simulink model "laneChange3"  (R2017a)
settings: Solver=VariableStepAuto  StartTime=0  StopTime=10  MaxStep=0.05  RelTol=1e-3
model workspace (MAT data in the model file):
  FARAWAY = Simulink.Parameter
  FARAWAY.Value = 100
  FARAWAY.DataType = 'auto'
  FARAWAY.Dimensions = [1 1]
  LANE_NUM = 2
  LANE_WIDTH = 1
  MIN_SAFE_DIST = Simulink.Parameter
  MIN_SAFE_DIST.Value = 1
  MIN_SAFE_DIST.DataType = 'auto'
  MIN_SAFE_DIST.Dimensions = [1 1]
  ROAD_WIDTH = 2
  SAFE_FACTOR = Simulink.Parameter
  SAFE_FACTOR.Value = 0.25
  SAFE_FACTOR.DataType = 'auto'
  SAFE_FACTOR.Dimensions = [1 1]
  WORLD_SIZE = 12
  dt = Simulink.Parameter
  dt.Value = 0.05
  dt.DataType = 'auto'
  dt.Dimensions = [1 1]
undefined symbols (not defined in the file or in its folder): m, n
(part 1 of 2)
settings Model: Creator=larry  LastModifiedBy=larry

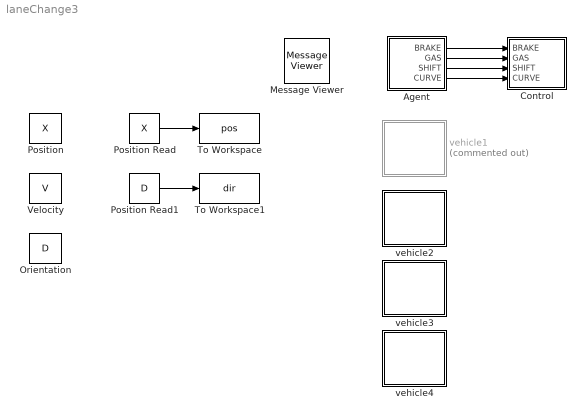
== system laneChange3 ==
  Agent : Stateflow chart  TreatAsAtomicUnit=on
  Control : Stateflow chart  TreatAsAtomicUnit=on
  Message Viewer : MessageViewer
  Orientation : DataStoreMemory  DataStoreName=D  WriteAfterReadMsg=warning  InitialValue=[1 1 1 1;0 0 0 0]  ShowAdditionalParam=off  OutDataTypeStr=double
  Position : DataStoreMemory  DataStoreName=X  InitialValue=[-11 -11 -9 11;-0.5 0.5 0.5 0.5]  ShowAdditionalParam=off  OutDataTypeStr=double
  Position Read : DataStoreRead  DataStoreName=X
  Position Read1 : DataStoreRead  DataStoreName=D
  To Workspace : ToWorkspace  VariableName=pos  SampleTime=-1
  To Workspace1 : ToWorkspace  VariableName=dir  SampleTime=-1
  Velocity : DataStoreMemory  DataStoreName=V  InitialValue=[0 0 0 0;0 0 0 0]  ShowAdditionalParam=off  OutDataTypeStr=double
  vehicle1 : Stateflow chart  Commented=on  TreatAsAtomicUnit=on
  vehicle2 : Stateflow chart  TreatAsAtomicUnit=on
  vehicle3 : Stateflow chart  TreatAsAtomicUnit=on
  vehicle4 : Stateflow chart  TreatAsAtomicUnit=on
  wires:
  Position Read/1 -> To Workspace/1
  Agent/2(GAS) -> Control/2(GAS)
  Agent/1(BRAKE) -> Control/1(BRAKE)
  Agent/3(SHIFT) -> Control/3(SHIFT)
  Agent/4(CURVE) -> Control/4(CURVE)
  Position Read1/1 -> To Workspace1/1

== stateflow chart laneChange3/vehicle2 ==
  state Straight
    en:
    safeDist = max(norm(V(:,this))*SAFE_FACTOR,MIN_SAFE_DIST);
    du:
    safeDist = max(norm(V(:,this))*SAFE_FACTOR,MIN_SAFE_DIST);
    state Follow
      en:
      [dxfr, dvfr] = frontCarInfo();
      du:
      [dxfr, dvfr] = frontCarInfo();
      state Safe
        du:
        if dvfr < 0
        accelerateDrive();
        else
        slowDownDrive();
        end
      state Dangerous
        du:
        slowDownDrive();
      Safe -> Dangerous : [dxfr < 1*safeDist]
      Dangerous -> Safe : [dxfr > 1.5*safeDist]
      (default) -> Dangerous [order 2]
      (default) -> Safe [order 1] : [dxfr > 1.5*safeDist]
    state FreeDriving
      state Accelerate
        du:
        accelerateDrive();
      state FixRate
        en:
        setRateTo(V_MAX);
        du:
        fixedRateDrive();
      (default) -> Accelerate [order 2]
      Accelerate -> FixRate : [reach(V_MAX)]
      (default) -> FixRate [order 1] : [reach(V_MAX)]
    (default) -> Follow [order 1] : [hasFrontCar()]
    (default) -> FreeDriving [order 2]
    FreeDriving -> Follow : [hasFrontCar()]
    Follow -> FreeDriving : [frontCarHasLeft()]
  data: res function_output; res function_output; res function_output; target function_input; target function_input; dx function_output; dv function_output; idx function_output; X data_store_memory; this local uint8 size=1 =uint8(2); A_MAX constant double =2.5; D data_store_memory; V_MAX constant double =1.5; V data_store_memory; MIN_SAFE_DIST parameter; WORLD_SIZE parameter; dt parameter; dxfr local; dvfr local; safeDist local; FARAWAY parameter; SAFE_FACTOR parameter
  function slowDownDrive:
    | function slowDownDrive
    |  
    | x = X(:,this);
    | v = V(:,this);
    | a = D(:,this) * (-A_MAX);
    | 
    | if isequal(v, [0;0])
    |     return;
    | end
    | 
    | x = x + v * dt + 0.5 * a * dt * dt;
    | if dot(v, v+a*dt) >= 0
    |     v = v + a * dt;
    | else
    |     v = 0 * v;
    | end
    | 
    | % a rounded world
    | if x(1) > WORLD_SIZE
    |     x(1) = -WORLD_SIZE;
    | elseif x(1) < -WORLD_SIZE
    |     x(1) = WORLD_SIZE;
    | elseif x(2) > WORLD_SIZE
    |     x(2) = -WORLD_SIZE;
    | elseif x(2) < -WORLD_SIZE
    |     x(2) = WORLD_SIZE;
    | end
    | 
    | X(:,this) = x;
    | V(:,this) = v;
  function res = hasFrontCar:
    | function res = hasFrontCar
    | 
    | % constants
    | THRES = 1.5 * safeDist;
    | RANGE = 2 * WORLD_SIZE;
    | 
    | res = false;
    | 
    | % row of X: coordinate, col of X: num of cars
    | num = size(X, 2);
    | if num == 1
    |     return;
    | end
    | 
    | dx = ones(num, 1)*FARAWAY;
    | x = X(:,this);
    | d = D(:,this);
    | carSize = [0.3; 0.4];
    | 
    | for k=1:length(dx)
    |     
    |     if k ~= this
    |         % compute difference
    |         xdelta = X(:,k) - x;
    |     
    |         % parallel and vertical distance
    |         delta_p = dot(xdelta, d);
    |         delta_v = norm(xdelta - (d * delta_p));
    |     
    |         % vertical distance is larger than car width
    |         if delta_v < carSize(1)
    |             dx(k) = delta_p;
    |       
    |             % a rounded world
    |             dx(k) = mod((dx(k)+RANGE), RANGE);
    |         end
    |     end
    | end
    | 
    | % set zero dX to a large enough value
    | closest = min(dx);
    | res = closest <= THRES;
  function res = frontCarHasLeft:
    | function res = frontCarHasLeft
    | 
    | % Constants 
    | THRES = 2.5 * safeDist;
    | RANGE = 2 * WORLD_SIZE;
    | 
    | % if only one car in the environment return directly
    | res = true;
    | num = size(X, 1);
    | if num == 1
    |     return;
    | end
    | 
    | % get the closet car index and its distance
    | dx = zeros(num, 1);
    | x = X(:,this);
    | d = D(:,this);
    | car_size = [0.3; 0.4];
    | 
    | for k=1:length(dx)
    |     
    |     xdelta = X(:,k) - x;
    |     xdelta_p = dot(xdelta, d);                  % parallel component
    |     xdelta_v = norm(xdelta - (d * xdelta_p));   % vertical component
    |     
    |     % when the vertical component is larger than the car width
    |     if xdelta_v < car_size(1)
    |         dx(k) = xdelta_p;
    |         % since we are in the round world, normalize the distance if the 
    |         % front car is behind us 
    |         % a rounded world
    |         dx(k) = mod((dx(k)+RANGE), RANGE);
    |     else
    |         dx(k) = FARAWAY;
    |     end
    | end
    | 
    | % set the zero dx to a large enough value for convenience
    | dx(dx == 0) = FARAWAY;
    | closest = min(dx);
    | res = closest > THRES;
  function res = reach(target):
    | function res = reach(target)
    | 
    | res = abs(target - norm(V(:,this))) < 0.125;
  function accelerateDrive:
    | function accelerateDrive
    | 
    | x = X(:,this);
    | v = V(:,this);
    | a = D(:,this) * A_MAX;
    | 
    | x = x + v * dt + 0.5 * a * dt * dt;
    | v = v + a * dt;
    | 
    | % a rounded world
    | if x(1) > WORLD_SIZE
    |     x(1) = -WORLD_SIZE;
    | elseif x(1) < -WORLD_SIZE
    |     x(1) = WORLD_SIZE;
    | elseif x(2) > WORLD_SIZE
    |     x(2) = -WORLD_SIZE;
    | elseif x(2) < -WORLD_SIZE
    |     x(2) = WORLD_SIZE;
    | end
    | 
    | X(:,this) = x;
    | V(:,this) = v;
  function fixedRateDrive:
    | function fixedRateDrive
    | 
    | x = X(:,this);
    | v = V(:,this);
    | 
    | % update new position
    | x = x + v * dt;
    | 
    | % a rounded world
    | if x(1) > WORLD_SIZE
    |     x(1) = -WORLD_SIZE;
    | elseif x(1) < -WORLD_SIZE
    |     x(1) = WORLD_SIZE;
    | elseif x(2) > WORLD_SIZE
    |     x(2) = -WORLD_SIZE;
    | elseif x(2) < -WORLD_SIZE
    |     x(2) = WORLD_SIZE;
    | end
    | 
    | X(:,this) = x;
  function setRateTo(target):
    | function setRateTo(target)
    | 
    | V(:,this) = D(:,this) * target;
  function [dx,dv] = frontCarInfo:
    | function [dx,dv] = frontCarInfo()
    | 
    | index = frontCarIndex();
    | 
    | x = X(:,this);
    | v = V(:,this);
    | d = D(:,this);
    | 
    | xfront = X(:,index);
    | vfront = V(:,index);
    | 
    | range = 2 * WORLD_SIZE;
    | 
    | dx = mod((dot(xfront - x, d)+range), range);
    | dv = dot(vfront-v, d);
    | 
    | end
  function idx = frontCarIndex:
    | function idx = frontCarIndex
    | 
    | RANGE = 2*WORLD_SIZE;
    | 
    | dx = ones(size(X, 2), 1)*FARAWAY;
    | x = X(:,this);
    | v = V(:,this);
    | d = D(:,this);
    | 
    | for k=1:length(dx)
    |     xk = X(:,k);
    |     if k ~= this && (abs(xk(2)-x(2)) < 1)
    |         dx(k) = dot(xk - x, d);
    |         dx(k) = mod((dx(k)+RANGE), RANGE);
    |     end
    | end
    | 
    | % set zero dx to a large enough value
    | [~, idx] = min(dx);
    | idx = uint8(idx);
    | 
    | end

== stateflow chart laneChange3/vehicle3 ==
  state Straight
    en:
    safeDist = max(norm(V(:,this))*SAFE_FACTOR,MIN_SAFE_DIST);
    du:
    safeDist = max(norm(V(:,this))*SAFE_FACTOR,MIN_SAFE_DIST);
    state Follow
      en:
      [dxfr, dvfr] = frontCarInfo();
      du:
      [dxfr, dvfr] = frontCarInfo();
      state Safe
        du:
        if dvfr < 0
        accelerateDrive();
        else
        slowDownDrive();
        end
      state Dangerous
        du:
        slowDownDrive();
      Safe -> Dangerous : [dxfr < 1*safeDist]
      Dangerous -> Safe : [dxfr > 1.5*safeDist]
      (default) -> Dangerous [order 2]
      (default) -> Safe [order 1] : [dxfr > 1.5*safeDist]
    state FreeDriving
      state Accelerate
        du:
        accelerateDrive();
      state FixRate
        en:
        setRateTo(V_MAX);
        du:
        fixedRateDrive();
      (default) -> Accelerate [order 2]
      Accelerate -> FixRate : [reach(V_MAX)]
      (default) -> FixRate [order 1] : [reach(V_MAX)]
    (default) -> Follow [order 1] : [hasFrontCar()]
    (default) -> FreeDriving [order 2]
    FreeDriving -> Follow : [hasFrontCar()]
    Follow -> FreeDriving : [frontCarHasLeft()]
  data: res function_output; res function_output; res function_output; target function_input; target function_input; dx function_output; dv function_output; idx function_output; X data_store_memory; this local uint8 size=1 =uint8(3); A_MAX constant double =2.5; D data_store_memory; V_MAX constant double =2; V data_store_memory; MIN_SAFE_DIST parameter; WORLD_SIZE parameter; dt parameter; dxfr local; dvfr local; safeDist local; FARAWAY parameter; SAFE_FACTOR parameter
  function slowDownDrive:
    | function slowDownDrive
    |  
    | x = X(:,this);
    | v = V(:,this);
    | a = D(:,this) * (-A_MAX);
    | 
    | x = x + v * dt + 0.5 * a * dt * dt;
    | if dot(v, v+a*dt) >= 0
    |     v = v + a * dt;
    | else
    |     v = 0 * v;
    | end
    | % a rounded world
    | if x(1) > WORLD_SIZE
    |     x(1) = -WORLD_SIZE;
    | elseif x(1) < -WORLD_SIZE
    |     x(1) = WORLD_SIZE;
    | elseif x(2) > WORLD_SIZE
    |     x(2) = -WORLD_SIZE;
    | elseif x(2) < -WORLD_SIZE
    |     x(2) = WORLD_SIZE;
    | end
    | 
    | X(:,this) = x;
    | V(:,this) = v;
  function res = hasFrontCar:
    | function res = hasFrontCar
    | 
    | % constants
    | THRES = 1.5 * safeDist;
    | RANGE = 2 * WORLD_SIZE;
    | 
    | res = false;
    | 
    | % row of X: coordinate, col of X: num of cars
    | num = size(X, 2);
    | if num == 1
    |     return;
    | end
    | 
    | dx = ones(num, 1)*FARAWAY;
    | x = X(:,this);
    | d = D(:,this);
    | carSize = [0.3; 0.4];
    | 
    | for k=1:length(dx)
    |     
    |     if k ~= this
    |         % compute difference
    |         xdelta = X(:,k) - x;
    |     
    |         % parallel and vertical distance
    |         delta_p = dot(xdelta, d);
    |         delta_v = norm(xdelta - (d * delta_p));
    |     
    |         % vertical distance is larger than car width
    |         if delta_v < carSize(1)
    |             dx(k) = delta_p;
    |       
    |             % a rounded world
    |             dx(k) = mod((dx(k)+RANGE), RANGE);
    |         end
    |     end
    | end
    | 
    | % set zero dX to a large enough value
    | closest = min(dx);
    | res = closest <= THRES;
  function res = frontCarHasLeft:
    | function res = frontCarHasLeft
    | 
    | % Constants 
    | THRES = 2.5 * safeDist;
    | RANGE = 2 * WORLD_SIZE;
    | 
    | % if only one car in the environment return directly
    | res = true;
    | num = size(X, 1);
    | if num == 1
    |     return;
    | end
    | 
    | % get the closet car index and its distance
    | dx = zeros(num, 1);
    | x = X(:,this);
    | d = D(:,this);
    | car_size = [0.3; 0.4];
    | 
    | for k=1:length(dx)
    |     
    |     xdelta = X(:,k) - x;
    |     xdelta_p = dot(xdelta, d);                  % parallel component
    |     xdelta_v = norm(xdelta - (d * xdelta_p));   % vertical component
    |     
    |     % when the vertical component is larger than the car width
    |     if xdelta_v < car_size(1)
    |         dx(k) = xdelta_p;
    |         % since we are in the round world, normalize the distance if the 
    |         % front car is behind us 
    |         % a rounded world
    |         dx(k) = mod((dx(k)+RANGE), RANGE);
    |     else
    |         dx(k) = FARAWAY;
    |     end
    | end
    | 
    | % set the zero dx to a large enough value for convenience
    | dx(dx == 0) = FARAWAY;
    | closest = min(dx);
    | res = closest > THRES;
  function res = reach(target):
    | function res = reach(target)
    | 
    | res = abs(target - norm(V(:,this))) < 0.125;
  function accelerateDrive:
    | function accelerateDrive
    | 
    | x = X(:,this);
    | v = V(:,this);
    | a = D(:,this) * A_MAX;
    | 
    | x = x + v * dt + 0.5 * a * dt * dt;
    | v = v + a * dt;
    | 
    | % a rounded world
    | if x(1) > WORLD_SIZE
    |     x(1) = -WORLD_SIZE;
    | elseif x(1) < -WORLD_SIZE
    |     x(1) = WORLD_SIZE;
    | elseif x(2) > WORLD_SIZE
    |     x(2) = -WORLD_SIZE;
    | elseif x(2) < -WORLD_SIZE
    |     x(2) = WORLD_SIZE;
    | end
    | 
    | X(:,this) = x;
    | V(:,this) = v;
  function fixedRateDrive:
    | function fixedRateDrive
    | 
    | x = X(:,this);
    | v = V(:,this);
    | 
    | % update new position
    | x = x + v * dt;
    | 
    | % a rounded world
    | if x(1) > WORLD_SIZE
    |     x(1) = -WORLD_SIZE;
    | elseif x(1) < -WORLD_SIZE
    |     x(1) = WORLD_SIZE;
    | elseif x(2) > WORLD_SIZE
    |     x(2) = -WORLD_SIZE;
    | elseif x(2) < -WORLD_SIZE
    |     x(2) = WORLD_SIZE;
    | end
    | 
    | X(:,this) = x;
  function setRateTo(target):
    | function setRateTo(target)
    | 
    | V(:,this) = D(:,this) * target;
  function [dx,dv] = frontCarInfo:
    | function [dx,dv] = frontCarInfo()
    | 
    | index = frontCarIndex();
    | 
    | x = X(:,this);
    | v = V(:,this);
    | d = D(:,this);
    | 
    | xfront = X(:,index);
    | vfront = V(:,index);
    | 
    | range = 2 * WORLD_SIZE;
    | 
    | dx = mod((dot(xfront - x, d)+range), range);
    | dv = dot(vfront-v, d);
    | 
    | end
  function idx = frontCarIndex:
    | function idx = frontCarIndex
    | 
    | RANGE = 2*WORLD_SIZE;
    | 
    | dx = ones(size(X, 2), 1)*FARAWAY;
    | x = X(:,this);
    | v = V(:,this);
    | d = D(:,this);
    | 
    | for k=1:length(dx)
    |     xk = X(:,k);
    |     if k ~= this && (abs(xk(2)-x(2)) < 1)
    |         dx(k) = dot(xk - x, d);
    |         dx(k) = mod((dx(k)+RANGE), RANGE);
    |     end
    | end
    | 
    | % set zero dx to a large enough value
    | [~, idx] = min(dx);
    | idx = uint8(idx);
    | 
    | end

== stateflow chart laneChange3/vehicle4 ==
  state Straight
    en:
    safeDist = max(norm(V(:,this))*SAFE_FACTOR,MIN_SAFE_DIST);
    du:
    safeDist = max(norm(V(:,this))*SAFE_FACTOR,MIN_SAFE_DIST);
    state Follow
      en:
      [dxfr, dvfr] = frontCarInfo();
      du:
      [dxfr, dvfr] = frontCarInfo();
      state Safe
        du:
        if dvfr < 0
        accelerateDrive();
        else
        slowDownDrive();
        end
      state Dangerous
        du:
        slowDownDrive();
      Safe -> Dangerous : [dxfr < 1.5*safeDist]
      Dangerous -> Safe : [dxfr > 1*safeDist]
      (default) -> Dangerous [order 2]
      (default) -> Safe [order 1] : [dxfr > 1.5*safeDist]
    state FreeDriving
      state Accelerate
        du:
        accelerateDrive();
      state FixRate
        en:
        setRateTo(V_MAX);
        du:
        fixedRateDrive();
      (default) -> Accelerate [order 2]
      Accelerate -> FixRate : [reach(V_MAX)]
      (default) -> FixRate [order 1] : [reach(V_MAX)]
    (default) -> Follow [order 1] : [hasFrontCar()]
    (default) -> FreeDriving [order 2]
    FreeDriving -> Follow : [hasFrontCar()]
    Follow -> FreeDriving : [frontCarHasLeft()]
  data: res function_output; res function_output; res function_output; target function_input; target function_input; dx function_output; dv function_output; idx function_output; X data_store_memory; this local uint8 size=1 =uint8(4); A_MAX constant double =2.5; D data_store_memory; V_MAX constant double =2; V data_store_memory; MIN_SAFE_DIST parameter; WORLD_SIZE parameter; dt parameter; dxfr local; dvfr local; safeDist local; FARAWAY parameter; SAFE_FACTOR parameter
  function slowDownDrive:
    | function slowDownDrive
    |  
    | x = X(:,this);
    | v = V(:,this);
    | a = D(:,this) * (-A_MAX);
    | 
    | x = x + v * dt + 0.5 * a * dt * dt;
    | if dot(v, v+a*dt) >= 0
    |     v = v + a * dt;
    | else
    |     v = 0 * v;
    | end
    | 
    | % a rounded world
    | if x(1) > WORLD_SIZE
    |     x(1) = -WORLD_SIZE;
    | elseif x(1) < -WORLD_SIZE
    |     x(1) = WORLD_SIZE;
    | elseif x(2) > WORLD_SIZE
    |     x(2) = -WORLD_SIZE;
    | elseif x(2) < -WORLD_SIZE
    |     x(2) = WORLD_SIZE;
    | end
    | 
    | X(:,this) = x;
    | V(:,this) = v;
  function res = hasFrontCar:
    | function res = hasFrontCar
    | 
    | % constants
    | THRES = 1.5 * safeDist;
    | RANGE = 2 * WORLD_SIZE;
    | 
    | res = false;
    | 
    | % row of X: coordinate, col of X: num of cars
    | num = size(X, 2);
    | if num == 1
    |     return;
    | end
    | 
    | dx = ones(num, 1)*FARAWAY;
    | x = X(:,this);
    | d = D(:,this);
    | carSize = [0.3; 0.4];
    | 
    | for k=1:length(dx)
    |     
    |     if k ~= this
    |         % compute difference
    |         xdelta = X(:,k) - x;
    |     
    |         % parallel and vertical distance
    |         delta_p = dot(xdelta, d);
    |         delta_v = norm(xdelta - (d * delta_p));
    |     
    |         % vertical distance is larger than car width
    |         if delta_v < carSize(1)
    |             dx(k) = delta_p;
    |       
    |             % a rounded world
    |             dx(k) = mod((dx(k)+RANGE), RANGE);
    |         end
    |     end
    | end
    | 
    | % set zero dX to a large enough value
    | closest = min(dx);
    | res = closest <= THRES;
  function res = frontCarHasLeft:
    | function res = frontCarHasLeft
    | 
    | % Constants 
    | THRES = 2.5 * safeDist;
    | RANGE = 2 * WORLD_SIZE;
    | 
    | % if only one car in the environment return directly
    | res = true;
    | num = size(X, 1);
    | if num == 1
    |     return;
    | end
    | 
    | % get the closet car index and its distance
    | dx = zeros(num, 1);
    | x = X(:,this);
    | d = D(:,this);
    | car_size = [0.3; 0.4];
    | 
    | for k=1:length(dx)
    |     
    |     xdelta = X(:,k) - x;
    |     xdelta_p = dot(xdelta, d);                  % parallel component
    |     xdelta_v = norm(xdelta - (d * xdelta_p));   % vertical component
    |     
    |     % when the vertical component is larger than the car width
    |     if xdelta_v < car_size(1)
    |         dx(k) = xdelta_p;
    |         % since we are in the round world, normalize the distance if the 
    |         % front car is behind us 
    |         % a rounded world
    |         dx(k) = mod((dx(k)+RANGE), RANGE);
    |     else
    |         dx(k) = FARAWAY;
    |     end
    | end
    | 
    | % set the zero dx to a large enough value for convenience
    | dx(dx == 0) = FARAWAY;
    | closest = min(dx);
    | res = closest > THRES;
  function res = reach(target):
    | function res = reach(target)
    | 
    | res = abs(target - norm(V(:,this))) < 0.125;
  function accelerateDrive:
    | function accelerateDrive
    | 
    | x = X(:,this);
    | v = V(:,this);
    | a = D(:,this) * A_MAX;
    | 
    | x = x + v * dt + 0.5 * a * dt * dt;
    | v = v + a * dt;
    | 
    | % a rounded world
    | if x(1) > WORLD_SIZE
    |     x(1) = -WORLD_SIZE;
    | elseif x(1) < -WORLD_SIZE
    |     x(1) = WORLD_SIZE;
    | elseif x(2) > WORLD_SIZE
    |     x(2) = -WORLD_SIZE;
    | elseif x(2) < -WORLD_SIZE
    |     x(2) = WORLD_SIZE;
    | end
    | 
    | X(:,this) = x;
    | V(:,this) = v;
  function fixedRateDrive:
    | function fixedRateDrive
    | 
    | x = X(:,this);
    | v = V(:,this);
    | 
    | % update new position
    | x = x + v * dt;
    | 
    | % a rounded world
    | if x(1) > WORLD_SIZE
    |     x(1) = -WORLD_SIZE;
    | elseif x(1) < -WORLD_SIZE
    |     x(1) = WORLD_SIZE;
    | elseif x(2) > WORLD_SIZE
    |     x(2) = -WORLD_SIZE;
    | elseif x(2) < -WORLD_SIZE
    |     x(2) = WORLD_SIZE;
    | end
    | 
    | X(:,this) = x;
  function setRateTo(target):
    | function setRateTo(target)
    | 
    | V(:,this) = D(:,this) * target;
  function [dx,dv] = frontCarInfo:
    | function [dx,dv] = frontCarInfo()
    | 
    | index = frontCarIndex();
    | 
    | x = X(:,this);
    | v = V(:,this);
    | d = D(:,this);
    | 
    | xfront = X(:,index);
    | vfront = V(:,index);
    | 
    | range = 2 * WORLD_SIZE;
    | 
    | dx = mod((dot(xfront - x, d)+range), range);
    | dv = dot(vfront-v, d);
    | 
    | end
  function idx = frontCarIndex:
    | function idx = frontCarIndex
    | 
    | RANGE = 2*WORLD_SIZE;
    | 
    | dx = ones(size(X, 2), 1)*FARAWAY;
    | x = X(:,this);
    | v = V(:,this);
    | d = D(:,this);
    | 
    | for k=1:length(dx)
    |     xk = X(:,k);
    |     if k ~= this && (abs(xk(2)-x(2)) < 1)
    |         dx(k) = dot(xk - x, d);
    |         dx(k) = mod((dx(k)+RANGE), RANGE);
    |     end
    | end
    | 
    | % set zero dx to a large enough value
    | [~, idx] = min(dx);
    | idx = uint8(idx);
    | 
    | end

== stateflow chart laneChange3/vehicle1 ==
  state Straight
    en:
    safeDist = max(norm(V(:,this))*1,MIN_SAFE_DIST);
    du:
    safeDist = max(norm(V(:,this))*1,MIN_SAFE_DIST);
    state FreeDriving
      state Accelerate
        du:
        accelerateDrive();
      state FixRate
        en:
        setRateTo(V_MAX);
        du:
        fixedRateDrive();
      (default) -> Accelerate [order 2]
      Accelerate -> FixRate : [higherThan(V_MAX)]
      (default) -> FixRate [order 1] : [higherThan(V_MAX)]
    state Follow
      en:
      [dxfr, dvfr] = frontCarInfo();
      du:
      [dxfr, dvfr] = frontCarInfo();
      state Safe
        du:
        if dvfr < 0
        accelerateDrive();
        elseif dvfr == 0
        fixedRateDrive();
        else
        slowDownDrive();
        end
      state Dangerous
        du:
        slowDownDrive();
      Safe -> Dangerous : [dxfr < 1*safeDist]
      Dangerous -> Safe : [dxfr > 1.5*safeDist]
      (default) -> Dangerous [order 2]
      (default) -> Safe [order 1] : [dxfr > 1.5*safeDist]
    (default) -> FreeDriving [order 2]
    (default) -> Follow [order 1] : [hasFrontCar()]
    FreeDriving -> Follow : [hasFrontCar()]
    Follow -> FreeDriving : [frontCarHasLeft()]
  state WaitToSwitchRight
    state SlowDown
      du:
      slowDownDrive();
    state fixedRate
      en:
      setRateTo(0.5*V_MAX);
      du:
      fixedRateDrive();
    (default) -> WaitToSwitchRight.SlowDown
    WaitToSwitchRight.SlowDown -> WaitToSwitchRight.fixedRate : [lowerThan(0.5*V_MAX)]
  state WaitToSwitchLeft
    state SlowDown
      du:
      slowDownDrive();
    state fixedRate
      en:
      setRateTo(0.5*V_MAX);
      du:
      fixedRateDrive();
    (default) -> WaitToSwitchLeft.SlowDown
    WaitToSwitchLeft.SlowDown -> WaitToSwitchLeft.fixedRate : [lowerThan(0.5*V_MAX)]
  state SwitchToLeftLane
    state ShiftLeft
      du:
      leftShiftDrive();
    state WaitDuringSwitchLeft
      du:
      fixedRateDrive();
    (default) -> ShiftLeft
    ShiftLeft -> WaitDuringSwitchLeft : [alwaysFalse()]
    WaitDuringSwitchLeft -> ShiftLeft : [alwaysFalse()]
  state SwitchToRightLane
    state SwitchRight
      du:
      rightShiftDrive();
    state WaitToSwitchRight
      du:
      fixedRateDrive();
    (default) -> SwitchRight
    SwitchRight -> SwitchToRightLane.WaitToSwitchRight : [alwaysFalse()]
    SwitchToRightLane.WaitToSwitchRight -> SwitchRight : [alwaysFalse()]
  (default) -> Straight
  SwitchToRightLane -> Straight [order 1] : [completeSwitchLane()]
      | {X(2,this) = yend;}
  WaitToSwitchRight -> Straight [order 2] : after(5, sec)
  (junction 130) -> Straight
  Straight -> (junction 128) : after(5, sec)
  WaitToSwitchLeft -> Straight [order 1] : after(5, sec)
  SwitchToLeftLane -> Straight [order 1] : [completeSwitchLane()]
      | {X(2,this) = yend;}
  (junction 128) -> (junction 130) [order 2]
  (junction 143) -> (junction 130) [order 3]
  (junction 128) -> (junction 143) [order 1] : [higherThan(0.5*V_MAX)]
  (junction 143) -> WaitToSwitchRight [order 2] : [decision == Decision.Right]
      | {prepareSwitchRight();}
  (junction 143) -> WaitToSwitchLeft [order 1] : [decision == Decision.Left &&...
      | hasLeftLane()]
      | {prepareSwitchLeft();}
  WaitToSwitchLeft -> SwitchToLeftLane [order 2] : [leftLaneClear()]
  WaitToSwitchRight -> SwitchToRightLane [order 1] : [rightLaneClear()]
  (junction 113) -> SwitchToRightLane [order 1] : [halfOnShift]
  SwitchToRightLane -> (junction 113) [order 2] : after(5,sec)
  (junction 113) -> SwitchToLeftLane [order 2]
  (junction 114) -> SwitchToRightLane [order 2]
  SwitchToLeftLane -> (junction 114) [order 2] : after(5, sec)
  (junction 114) -> SwitchToLeftLane [order 1] : [halfOnShift]
  data: target function_input; res function_output; res function_output; res function_output; res function_output; target function_input; target function_input; dx function_output; dv function_output; idx function_output; res function_output; res function_output; res function_output; res function_output; res function_output; res function_output; X data_store_memory; this local uint8 size=1 =uint8(1); A_MAX constant double =2.5; D data_store_memory; V_MAX constant double =2.5; V data_store_memory; MIN_SAFE_DIST parameter; WORLD_SIZE parameter; dt parameter; dxfr local; dvfr local; safeDist local; FARAWAY parameter; yend local; ystart local; LANE_NUM parameter; ROAD_WIDTH parameter; decision local Enum: Decision =Decision.Left
  function res = lowerThan(target):
    | function res = lowerThan(target)
    |  
    | v_norm = norm(V(:,this));
    | 
    | res = (v_norm <= target) || ((norm(V(:,this))-target) < 0.125);
  function slowDownDrive:
    | function slowDownDrive
    |  
    | x = X(:,this);
    | v = V(:,this);
    | a = D(:,this) * (-A_MAX);
    | 
    | x = x + v * dt + 0.5 * a * dt * dt;
    | v = v + a * dt;
    | 
    | % a rounded world
    | if x(1) > WORLD_SIZE
    |     x(1) = -WORLD_SIZE;
    | elseif x(1) < -WORLD_SIZE
    |     x(1) = WORLD_SIZE;
    | elseif x(2) > WORLD_SIZE
    |     x(2) = -WORLD_SIZE;
    | elseif x(2) < -WORLD_SIZE
    |     x(2) = WORLD_SIZE;
    | end
    | 
    | X(:,this) = x;
    | V(:,this) = v;
  function res = hasFrontCar:
    | function res = hasFrontCar
    | 
    | % constants
    | THRES = 1.5 * safeDist;
    | RANGE = 2 * WORLD_SIZE;
    | 
    | res = false;
    | 
    | % row of X: coordinate, col of X: num of cars
    | num = size(X, 2);
    | if num == 1
    |     return;
    | end
    | 
    | dx = ones(num, 1)*FARAWAY;
    | x = X(:,this);
    | d = D(:,this);
    | carSize = [0.3; 0.4];
    | 
    | for k=1:length(dx)
    |     
    |     if k ~= this
    |         % compute difference
    |         xdelta = X(:,k) - x;
    |     
    |         % parallel and vertical distance
    |         delta_p = dot(xdelta, d);
    |         delta_v = norm(xdelta - (d * delta_p));
    |     
    |         % vertical distance is larger than car width
    |         if delta_v < carSize(1)
    |             dx(k) = delta_p;
    |       
    |             % a rounded world
    |             dx(k) = mod((dx(k)+RANGE), RANGE);
    |         end
    |     end
    | end
    | 
    | % set zero dX to a large enough value
    | closest = min(dx);
    | res = closest <= THRES;
  function res = frontCarHasLeft:
    | function res = frontCarHasLeft
    | 
    | % Constants 
    | THRES = 2 * safeDist;
    | RANGE = 2 * WORLD_SIZE;
    | 
    | % if only one car in the environment return directly
    | res = true;
    | num = size(X, 1);
    | if num == 1
    |     return;
    | end
    | 
    | % get the closet car index and its distance
    | dx = zeros(num, 1);
    | x = X(:,this);
    | d = D(:,this);
    | car_size = [0.3; 0.4];
    | 
    | for k=1:length(dx)
    |     
    |     xdelta = X(:,k) - x;
    |     xdelta_p = dot(xdelta, d);                  % parallel component
    |     xdelta_v = norm(xdelta - (d * xdelta_p));   % vertical component
    |     
    |     % when the vertical component is larger than the car width
    |     if xdelta_v < car_size(1)
    |         dx(k) = xdelta_p;
    |         % since we are in the round world, normalize the distance if the 
    |         % front car is behind us 
    |         % a rounded world
    |         dx(k) = mod((dx(k)+RANGE), RANGE);
    |     else
    |         dx(k) = FARAWAY;
    |     end
    | end
    | 
    | % set the zero dx to a large enough value for convenience
    | dx(dx == 0) = FARAWAY;
    | closest = min(dx);
    | res = closest > THRES;
  function res = higherThan(target):
    | function res = higherThan(target)
    | 
    | v_norm = norm(V(:,this));
    | 
    | res = (v_norm >= target) || ((target - norm(V(:,this))) < 0.125);
  function accelerateDrive:
    | function accelerateDrive
    | 
    | x = X(:,this);
    | v = V(:,this);
    | a = D(:,this) * A_MAX;
    | 
    | x = x + v * dt + 0.5 * a * dt * dt;
    | v = v + a * dt;
    | 
    | % a rounded world
    | if x(1) > WORLD_SIZE
    |     x(1) = -WORLD_SIZE;
    | elseif x(1) < -WORLD_SIZE
    |     x(1) = WORLD_SIZE;
    | elseif x(2) > WORLD_SIZE
    |     x(2) = -WORLD_SIZE;
    | elseif x(2) < -WORLD_SIZE
    |     x(2) = WORLD_SIZE;
    | end
    | 
    | X(:,this) = x;
    | V(:,this) = v;
  function fixedRateDrive:
    | function fixedRateDrive
    | 
    | x = X(:,this);
    | v = V(:,this);
    | 
    | % update new position
    | x = x + v * dt;
    | 
    | % a rounded world
    | if x(1) > WORLD_SIZE
    |     x(1) = -WORLD_SIZE;
    | elseif x(1) < -WORLD_SIZE
    |     x(1) = WORLD_SIZE;
    | elseif x(2) > WORLD_SIZE
    |     x(2) = -WORLD_SIZE;
    | elseif x(2) < -WORLD_SIZE
    |     x(2) = WORLD_SIZE;
    | end
    | 
    | X(:,this) = x;
  function setRateTo(target):
    | function setRateTo(target)
    | 
    | V(:,this) = D(:,this) * target;
  function [dx,dv] = frontCarInfo:
    | function [dx,dv] = frontCarInfo()
    | 
    | index = frontCarIndex();
    | 
    | x = X(:,this);
    | v = V(:,this);
    | d = D(:,this);
    | 
    | xfront = X(:,index);
    | vfront = V(:,index);
    | 
    | range = 2 * WORLD_SIZE;
    | 
    | dx = mod((dot(xfront - x, d)+range), range);
    | dv = dot(vfront-v, d);
    | 
    | end
  function idx = frontCarIndex:
    | function idx = frontCarIndex
    | 
    | RANGE = 2*WORLD_SIZE;
    | 
    | dx = ones(size(X, 2), 1)*FARAWAY;
    | x = X(:,this);
    | v = V(:,this);
    | d = D(:,this);
    | 
    | for k=1:length(dx)
    |     xk = X(:,k);
    |     if k ~= this && (abs(xk(2)-x(2)) < 1)
    |         dx(k) = dot(xk - x, d);
    |         dx(k) = mod((dx(k)+RANGE), RANGE);
    |     end
    | end
    | 
    | % set zero dx to a large enough value
    | [~, idx] = min(dx);
    | idx = uint8(idx);
    | 
    | end
  function res = rightLaneClear:
    | function res = rightLaneClear
    | 
    | res = true;
    | 
    | lnum = LANE_NUM;
    | rwidth = ROAD_WIDTH;
    | range = 2*WORLD_SIZE;
    | 
    | x = X(:,this);
    | v = V(:,this);
    | 
    | pos_y = FARAWAY*ones(20, 1);
    | if mod(lnum,2) == 0
    |     k = (-1*(rwidth/2-0.5));
    |     for i=1:lnum
    |         pos_y(i) = k;
    |         k = k + 1;
    |     end
    | else
    |     k = (-1*(rwidth/2));
    |     for i=1:lnum
    |         pos_y(i) = k;
    |         k = k + 1;
    |     end
    | end
    | 
    | [~, index] = min(abs(pos_y-x(2)));
    | if index == 1
    |     res = false;
    |     
    |     % TODO: change the planning to demo different scenario
    |     
    |     return;
    | end
    | 
    | ys = X(2,:)-x(2);
    | ys(this) = FARAWAY;
    | indices = find(ys < 0 & ys >= -1);  
    | if isempty(indices)
    |     return;
    | end
    | 
    | for i = 1:length(indices)
    |     
    |     idx = indices(i);
    |     xb = X(:,idx);
    |     vb = V(:,idx);
    |     
    |     dx = mod(x(1)+range-xb(1), range);
    |     dv = v(1) - vb(1);
    |     
    |     backSafeDist = max(1*vb(1), MIN_SAFE_DIST);
    | 
    |     % front car 
    |     if dx >= range - 0.5*safeDist
    |         res = false;
    |     % the car in the behind is too close
    |     elseif dx <= backSafeDist
    |         res = false;
    |     % the distance is larger than safeDist but current speed is too slow
    |     elseif dx <= 1.5*backSafeDist && dv < 0
    |         disp(1.5*backSafeDist);
    |         res = false;
    |     end
    | end
  function prepareSwitchRight:
    | function prepareSwitchRight
    | 
    | x = X(:,this);
    | 
    | ystart = x(2);
    | yend = x(2)-1;
  function prepareSwitchLeft:
    | function prepareSwitchLeft
    |  
    | x = X(:,this);
    | 
    | ystart = x(2);
    | yend = x(2)+1;
  function rightShiftDrive:
    | function rightShiftDrive
    |  
    | x = X(:,this);
    | v = V(:,this);
    | 
    | % update new position
    | x = x + v * dt;
    | dy = (yend-ystart)/20;
    | dp = [0; dy];
    | x = x + dp;
    | 
    | % a rounded world
    | if x(1) > WORLD_SIZE
    |     x(1) = -WORLD_SIZE;
    | elseif x(1) < -WORLD_SIZE
    |     x(1) = WORLD_SIZE;
    | elseif x(2) > WORLD_SIZE
    |     x(2) = -WORLD_SIZE;
    | elseif x(2) < -WORLD_SIZE
    |     x(2) = WORLD_SIZE;
    | end
    | 
    | X(:,this) = x;
  function leftShiftDrive:
    | function leftShiftDrive
    |  
    | x = X(:,this);
    | v = V(:,this);
    | 
    | % update new position
    | x = x + v * dt;
    | dy = (yend-ystart)/20;
    | dp = [0; dy];
    | x = x + dp;
    | 
    | % a rounded world
    | if x(1) > WORLD_SIZE
    |     x(1) = -WORLD_SIZE;
    | elseif x(1) < -WORLD_SIZE
    |     x(1) = WORLD_SIZE;
    | elseif x(2) > WORLD_SIZE
    |     x(2) = -WORLD_SIZE;
    | elseif x(2) < -WORLD_SIZE
    |     x(2) = WORLD_SIZE;
    | end
    | 
    | X(:,this) = x;
  function res = completeSwitchLane:
    | function res = completeSwitchLane
    |  
    | x = X(:,this);
    | 
    | res = abs(yend - x(2)) <= 0.05;
  function res = leftLaneClear:
    | function res = leftLaneClear
    |  
    | res = true;
    | 
    | lnum = LANE_NUM;
    | rwidth = ROAD_WIDTH;
    | range = 2*WORLD_SIZE;
    | 
    | x = X(:,this);
    | v = V(:,this);
    | 
    | pos_y = FARAWAY*ones(20, 1);
    | if mod(lnum,2) == 0
    |     k = (-1*(rwidth/2-0.5));
    |     for i=1:lnum
    |         pos_y(i) = k;
    |         k = k + 1;
    |     end
    | else
    |     k = (-1*(rwidth/2));
    |     for i=1:lnum
    |         pos_y(i) = k;
    |         k = k + 1;
    |     end
    | end
    | 
    | [~, index] = min(abs(pos_y-x(2)));
    | if index == lnum
    |     res = false;
    |     
    |     % TODO: change the planning to demo different scenario
    |     
    |     return;
    | end
    | 
    | ys = X(2,:)-x(2);
    | ys(this) = FARAWAY;
    | indices = find(ys > 0 & ys <= 1);  
    | if isempty(indices)
    |     return;
    | end
    | 
    | for i = 1:length(indices)
    |     
    |     idx = indices(i);
    |     xb = X(:,idx);
    |     vb = V(:,idx);
    |     
    |     dx = mod(x(1)+range-xb(1), range);
    |     dv = v(1) - vb(1);
    |     
    |     backSafeDist = max(1*vb(1), MIN_SAFE_DIST);
    | 
    |     % front car 
    |     if dx >= range - 0.5*safeDist
    |         res = false;
    |     % the car in the behind is too close
    |     elseif dx <= backSafeDist
    |         res = false;
    |     % the distance is larger than safeDist but current speed is too slow
    |     elseif dx <= 1.5*backSafeDist && dv < 0
    |         disp(1.5*backSafeDist);
    |         res = false;
    |     end
    | end
  function res = halfOnShift:
    | function res = halfOnShift
    | 
    | res = false;
  function res = alwaysFalse:
    | function res = alwaysFalse
    | 
    | res = false;
  function res = hasLeftLane:
    | function res = hasLeftLane
    | 
    | res = true;
    | 
    | lnum = LANE_NUM;
    | rwidth = ROAD_WIDTH;
    | range = 2*WORLD_SIZE;
    | 
    | x = X(:,this);
    | v = V(:,this);
    | 
    | pos_y = FARAWAY*ones(20, 1);
    | if mod(lnum,2) == 0
    |     k = (-1*(rwidth/2-0.5));
    |     for i=1:lnum
    |         pos_y(i) = k;
    |         k = k + 1;
    |     end
    | else
    |     k = (-1*(rwidth/2));
    |     for i=1:lnum
    |         pos_y(i) = k;
    |         k = k + 1;
    |     end
    | end
    | 
    | [~, index] = min(abs(pos_y-x(2)));
    | if index == lnum
    |     res = false;
    | end

== stateflow chart laneChange3/Control ==
  state Straight
    state SlowToStop
      state Stop
      state SlowToTarget
        en:
        target = msg(1);
        du:
        slowDownDrive;
      state Transition
      (default) -> Stop [order 1] : [isStopped]
      Stop -> Stop : [needSlowDown]
      SlowToTarget -> SlowToTarget [order 2] : [needSlowDown]
      (default) -> (junction 112) [order 2]
      (junction 112) -> Stop [order 1] : [isStopped]
      SlowToTarget -> (junction 112) [order 1] : [lowerThan(target)]
          | {setRateTo(target);}
      (junction 112) -> Transition [order 2]
    state AccToTarget
      state Acc
        en:
        target = msg(1);
        du:
        accelerateDrive
      state FixedRate
        du:
        fixedRateDrive
      FixedRate -> Acc : [needSpeedUp]
      Acc -> Acc [order 2] : [needSpeedUp]
      Acc -> FixedRate [order 1] : [higherThan(target)]
          | {setRateTo(target);}
      (default) -> FixedRate
    (default) -> SlowToStop
    AccToTarget -> SlowToTarget : [needSlowDown]
    Transition -> FixedRate
    SlowToStop -> Acc : [needSpeedUp]
  state Drift
    en:
    yend = msg(1);
    ystart = msg(2);
    du:
    shiftDrive;
  state res = needSlowDown [function]
    (default) -> (junction 23) : {msg = zeros(2,1);
        | res = false;}
    (junction 23) -> (junction 22) [order 1] : BRAKE
    (junction 22) -> (junction 24) : {msg = BRAKE.data;
        | TRASH.data = BRAKE.data;
        | forward(BRAKE,TRASH);}
    (junction 24) -> (junction 23) : {res = true;}
    (junction 23) -> (junction 25) [order 2]
  state res = needSpeedUp [function]
    (default) -> (junction 39) : {msg = zeros(2,1);
        | res = false;}
    (junction 39) -> (junction 38) [order 1] : GAS
    (junction 38) -> (junction 40) : {msg = GAS.data;
        | TRASH.data = GAS.data;
        | forward(GAS,TRASH);}
    (junction 40) -> (junction 39) : {res = true;}
    (junction 39) -> (junction 41) [order 2]
  state Curve
    en:
    pf = msg(1:2);
    du:
    curveDrive(pf, [1;0]);
    ex:
    D(:,this) = [1;0];
    V(:,this) = [1;0]*V_MAX;
  state res = needShift [function]
    (default) -> (junction 69) : {msg = zeros(2,1);
        | res = false;}
    (junction 69) -> (junction 68) [order 1] : SHIFT
    (junction 68) -> (junction 70) : {msg = SHIFT.data;
        | TRASH.data = SHIFT.data;
        | forward(SHIFT,TRASH);}
    (junction 70) -> (junction 69) : {res = true;}
    (junction 69) -> (junction 71) [order 2]
  state res = wantCurveDrive [function]
    (default) -> (junction 157) : {msg = zeros(2,1);
        | res = false;}
    (junction 157) -> (junction 156) [order 1] : CURVE
    (junction 156) -> (junction 159) : {msg = CURVE.data;
        | TRASH.data = CURVE.data;
        | forward(CURVE,TRASH);}
    (junction 159) -> (junction 157) : {res = true;}
    (junction 157) -> (junction 158) [order 2]
  (default) -> Straight
  Drift -> SlowToTarget [order 1] : [needSlowDown]
  Straight -> Drift [order 1] : [needShift]
  Drift -> Straight [order 2] : [shiftCompleted]
  Straight -> Curve [order 2] : [wantCurveDrive]
  Curve -> Straight : [completeBezierMove(pf)]
  data: p0 function_input; d0 function_input; p2 function_input; d2 function_input; res function_output; p_mid function_output; p2 function_input double size=[2 1]; d2 function_input double size=[2 1]; res function_output; p2 function_input double; d2 function_input double size=[2 1]; res function_output double size=1; p0 function_input double size=[2 1]; p1 function_input double size=[2 1]; p2 function_input double size=[2 1]; res function_output; p2 function_input; res function_output; rate function_input; res function_output; rate function_input; res function_output; rate function_input; res function_output; target local; res function_output; res function_output; res function_output; res function_output; this local uint8 =uint8(1); TRASH local; msg local size=[2 1]; V data_store_memory; A_MAX constant double =2.5; WORLD_SIZE parameter; BRAKE input; GAS input; SHIFT input; X data_store_memory; D data_store_memory; yend local; ystart local; dt parameter; DY_SHIFT constant double =0.0625; pf local; V_MIN constant double =0.125; CURVE input double; V_MAX constant double =1.75
  function [res, p_mid] = intersection(p0, d0, p2, d2):
    | function [res, p_mid] = intersection(p0, d0, p2, d2)
    | 
    | res = true;
    | p_mid = (p0 + p2)/2;
    | 
    | 
    | % xi = p0(1);
    | % yi = p0(2);
    | % ai = d0(1);
    | % bi = d0(2);
    | % xf = p2(1);
    | % yf = p2(2);
    | % af = d2(1);
    | % bf = d2(2);
    | % 
    | % assert(norm(d0) ~= 0 && norm(d2) ~= 0);
    | % 
    | % p_mid = p0;
    | % 
    | % dp = p2 - p0;
    | % dp_norm = norm(dp);
    | % if dp_norm == 0
    | %     disp('pi and pf are overlapped');
    | %     res = true;
    | %     return;
    | % end
    | % 
    | % dp = dp/dp_norm;
    | % if bi == 0
    | %     if bf == 0
    | %         if isequal(dp, [ai/abs(ai); 0])
    | %             res = true;
    | %             p_mid = (p0 + p2)/2;
    | %         else
    | %             res = true;
    | %             p_mid = (p0 + p2)/2;
    | %         end
    | %     else
    | %         tf = (yi - yf)/bf;
    | %         res = true;
    | %         p_mid = [xf + af*tf; yf + bf*tf];
    | %     end
    | % else
    | %     denominator = af*bi - ai*bf;
    | %     if denominator == 0
    | %         % the d0 and d2 are in parallel
    | %         d0 = d0/norm(d0);
    | %         if isequal(dp, d0)
    | %             res = true;
    | %             p_mid = (p0+p2)/2;
    | %         else
    | %             res = false;
    | %         end
    | %     else
    | %         res = true;
    | %         tf = ((bi*xi-ai*yi) - (bi*xf - ai*yf))/denominator;
    | %         p_mid = [xf + af*tf; yf + bf*tf];
    | %     end
    | % end
  function res = computeBezier2(p2, d2):
    | function res = computeBezier2(p2, d2)
    | 
    | p0 = X(:,this);
    | d0 = D(:,this);
    | 
    | % pf and df will be determined by a high level logic
    | [check, res] = intersection(p0, d0, p2, d2);
    | 
    | % assert(check, '[ASSERT] The check is supposed to be true');
  function curveDrive(p2, d2):
    | function curveDrive(p2, d2)
    | 
    | % d0 = D(:,this)
    | % d2
    | 
    | p0 = X(:,this);
    | p1 = computeBezier2(p2, d2);
    | % p2
    | 
    | th = dthNext(p0, p1, p2);
    | 
    | q0 = p0 * (1-th) + p1 * th;
    | q1 = p1 * (1-th) + p2 * th;
    | 
    | d = q1 - q0;
    | d = d/norm(d);
    | D(:,this) = d;
    | 
    | p = (1 - 2*th + th*th) * p0 + (2*th - 2*th*th) * p1 + (th*th)* p2;
    | dx = p - p0;
    | v = d*norm(dx)/dt;
    | 
    | X(:,this) = p;
    | V(:,this) = v;
  function res = dthNext(p0, p1, p2):
    | function res = dthNext(p0, p1, p2)
    | 
    | v = V(:,this);
    | v_norm = norm(v);
    | 
    | last = p0;
    | length = 0;
    | for i=0:0.01:1
    |     p = (1 - 2*i + i*i) * p0 + (2*i - 2*i*i) * p1 + (i*i)* p2;
    |     length = length + norm(p - last);
    |     last = p;
    | end
    | 
    | if v_norm > 0
    |     dist = dt*v_norm;
    |     if dist < length
    |         res = dist/length;
    |     else
    |         res = 1;
    |     end
    | else
    |     dist = dt*V_MIN;
    |     if dist < length
    |         res = dist/length;
    |     else
    |         res = 1;
    |     end
    | end
  function res = completeBezierMove(p2):
    | function res = completeBezierMove(p2)
    | 
    | % res = isequal(X(:,this), p2);
    | res = norm(abs(X(:,this)-p2)) < 0.05;
  function res = isStopped:
    | function res = isStopped
    |  
    | res = (norm(V(:,this)) < 0.125);
  function shiftDrive:
    | function shiftDrive
    |  
    | x = X(:,this);
    | v = V(:,this);
    | 
    | % calculate the shift distance
    | dy = yend - x(2);
    | if dy >= 0
    |     dy = min(DY_SHIFT, dy);
    | else
    |     dy = max(-DY_SHIFT, dy);
    | end
    | 
    | % calculate the overall move
    | dx = [0; dy];
    | x = x + dx + v * dt;
    | 
    | % a rounded world
    | if x(1) > WORLD_SIZE
    |     x(1) = -WORLD_SIZE;
    | elseif x(1) < -WORLD_SIZE
    |     x(1) = WORLD_SIZE;
    | elseif x(2) > WORLD_SIZE
    |     x(2) = -WORLD_SIZE;
    | elseif x(2) < -WORLD_SIZE
    |     x(2) = WORLD_SIZE;
    | end
    | 
    | % update next position
    | X(:,this) = x;
  function setRateTo(rate):
    | function setRateTo(rate)
    | 
    | V(:,this) = D(:,this) * rate;
  function res = shiftCompleted:
    | function res = shiftCompleted
    | 
    | x = X(:,this);
    | 
    | res = abs(x(2) - yend) == 0;
  function res = higherThan(rate):
    | function res = higherThan(rate)
    | 
    | v_norm = norm(V(:,this));
    | res = (v_norm >= rate) || ((rate - v_norm) < 0.125);
  function accelerateDrive:
    | function accelerateDrive
    | 
    | x = X(:,this);
    | v = V(:,this);
    | a = D(:,this) * A_MAX;
    | 
    | x = x + v * dt + 0.5 * a * dt * dt;
    | v = v + a * dt;
    | 
    | % a rounded world
    | if x(1) > WORLD_SIZE
    |     x(1) = -WORLD_SIZE;
    | elseif x(1) < -WORLD_SIZE
    |     x(1) = WORLD_SIZE;
    | elseif x(2) > WORLD_SIZE
    |     x(2) = -WORLD_SIZE;
    | elseif x(2) < -WORLD_SIZE
    |     x(2) = WORLD_SIZE;
    | end
    | 
    | X(:,this) = x;
    | V(:,this) = v;
  function res = lowerThan(rate):
    | function res = lowerThan(rate)
    |  
    | v_norm = norm(V(:,this));
    | res = (v_norm <= rate) || ((v_norm - rate) < 0.125);
  function fixedRateDrive:
    | function fixedRateDrive
    | 
    | x = X(:,this);
    | v = V(:,this);
    | 
    | % update new position
    | x = x + v * dt;
    | 
    | % a rounded world
    | if x(1) > WORLD_SIZE
    |     x(1) = -WORLD_SIZE;
    | elseif x(1) < -WORLD_SIZE
    |     x(1) = WORLD_SIZE;
    | elseif x(2) > WORLD_SIZE
    |     x(2) = -WORLD_SIZE;
    | elseif x(2) < -WORLD_SIZE
    |     x(2) = WORLD_SIZE;
    | end
    | 
    | X(:,this) = x;
  function slowDownDrive:
    | function slowDownDrive
    |  
    | x = X(:,this);
    | v = V(:,this);
    | a = D(:,this) * (-A_MAX);
    | 
    | x = x + v * dt + 0.5 * a * dt * dt;
    | v = v + a * dt;
    | 
    | % a rounded world
    | if x(1) > WORLD_SIZE
    |     x(1) = -WORLD_SIZE;
    | elseif x(1) < -WORLD_SIZE
    |     x(1) = WORLD_SIZE;
    | elseif x(2) > WORLD_SIZE
    |     x(2) = -WORLD_SIZE;
    | elseif x(2) < -WORLD_SIZE
    |     x(2) = WORLD_SIZE;
    | end
    | 
    | X(:,this) = x;
    | V(:,this) = v;
